simulink model "model"  (R2019b)
settings: Solver=VariableStepAuto  StartTime=0.0  StopTime=100  RelTol=1e-3
values from neighbouring files (symbols this model uses):
  a1 = 0.1    [start.m]
  a2 = 0.2    [start.m]
  b1 = 0.05    [start.m]
  b2 = 0.15    [start.m]
  En = 0.9284766909    [start.m]
  g = 0.03    [start.m]
  Kn = 0.01313064329    [start.m]
  Kxi = 0.014142    [start.m]
  Tn = 0.04642383454    [start.m]
  tstep = 1    [start.m]
  Txi = 0.1    [start.m]
  x0 = 1    [start.m]
  y0 = 1    [start.m]
libraries: simulink x2
settings Model: Creator=Roman  LastModifiedBy=romak

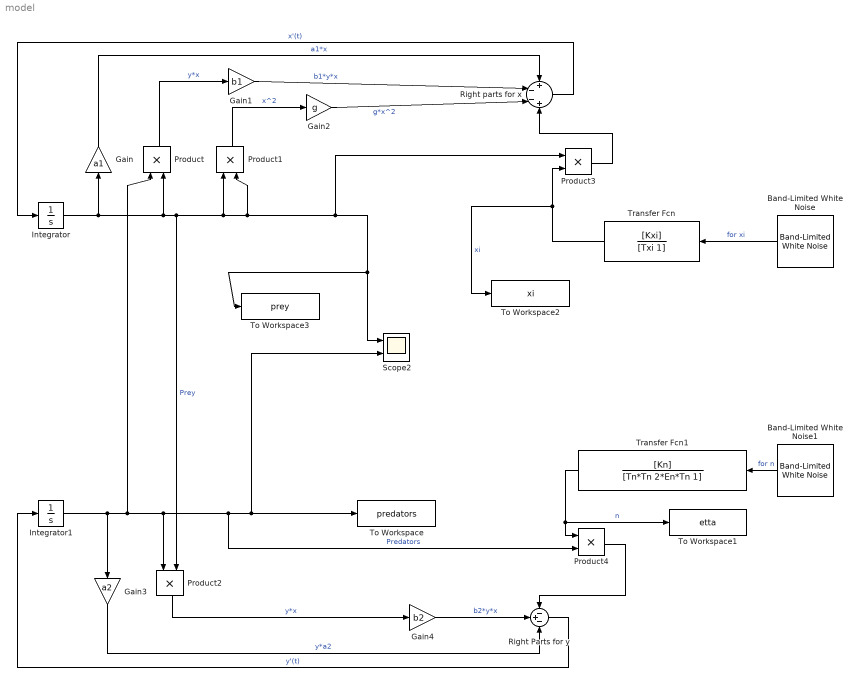
== system model ==
  Band-Limited White Noise : simulink/Sources/Band-Limited White Noise  Cov=[1]  Ts=tstep  seed=[1]
  Band-Limited White Noise1 : simulink/Sources/Band-Limited White Noise  Cov=[1]  Ts=tstep  seed=[2]
  Gain : Gain  Gain=a1
  Gain1 : Gain  Gain=b1
  Gain2 : Gain  Gain=g
  Gain3 : Gain  Gain=a2
  Gain4 : Gain  Gain=b2
  Integrator : Integrator  InitialCondition=x0
  Integrator1 : Integrator  InitialCondition=y0
  Product{,1..4} (5 alike) : Product
  "Right Parts for y " : Sum  Inputs=-+-
  Right parts for x : Sum  Inputs=+--+
  Scope2 : Scope  NumInputPorts=2
  To Workspace : ToWorkspace  VariableName=predators  SaveFormat=Timeseries  SampleTime=-1
  To Workspace1 : ToWorkspace  VariableName=etta  SaveFormat=Timeseries  SampleTime=-1
  To Workspace2 : ToWorkspace  VariableName=xi  SaveFormat=Timeseries  SampleTime=-1
  To Workspace3 : ToWorkspace  VariableName=prey  SaveFormat=Timeseries  SampleTime=-1
  Transfer Fcn : TransferFcn  Numerator=[Kxi]  Denominator=[Txi 1]
  Transfer Fcn1 : TransferFcn  Numerator=[Kn]  Denominator=[Tn*Tn 2*En*Tn 1]
  wires:
  Band-Limited White Noise/1 -> Transfer Fcn/1  "for xi"
  Band-Limited White Noise1/1 -> Transfer Fcn1/1  "for n"
  Transfer Fcn/1 -> To Workspace2/1, Product3/2  "xi"
  Transfer Fcn1/1 -> To Workspace1/1, Product4/1  "n"
  Integrator/1 -> Gain/1, Product1/1, Product3/1, Scope2/1, To Workspace3/1, Product1/2, Product2/2, Product/2  "Prey"
  Right parts for x/1 -> Integrator/1  "x'(t)"
  Gain/1 -> Right parts for x/1  "a1*x"
  Integrator1/1 -> Product4/2, Scope2/2, To Workspace/1, Product2/1, Product/1, Gain3/1  "Predators"
  Product/1 -> Gain1/1  "y*x"
  Gain1/1 -> Right parts for x/2  "b1*y*x"
  Product1/1 -> Gain2/1  "x^2"
  Gain2/1 -> Right parts for x/3  "g*x^2"
  Gain3/1 -> "Right Parts for y "/3  "y*a2"
  Product2/1 -> Gain4/1  "y*x"
  "Right Parts for y "/1 -> Integrator1/1  "y'(t)"
  Gain4/1 -> "Right Parts for y "/2  "b2*y*x"
  Product3/1 -> Right parts for x/4
  Product4/1 -> "Right Parts for y "/1
